simulink model "Sampling_switch_uncertainty"  (R2021b)
settings: Solver=VariableStepAuto  StartTime=0.0  StopTime=10.0  RelTol=1e-3
values from neighbouring files (symbols this model uses):
  bits_number = 13    [launch_pipeline_switch.m]
  cst = 2*pi*fin/1000    [launch_pipeline_switch.m]
  fin = antismear(fin_pre,fs,nfft)    [launch_pipeline_switch.m]
  ts = 1/fs    (= 1)    [launch_pipeline_switch.m]
(part 2 of 2)

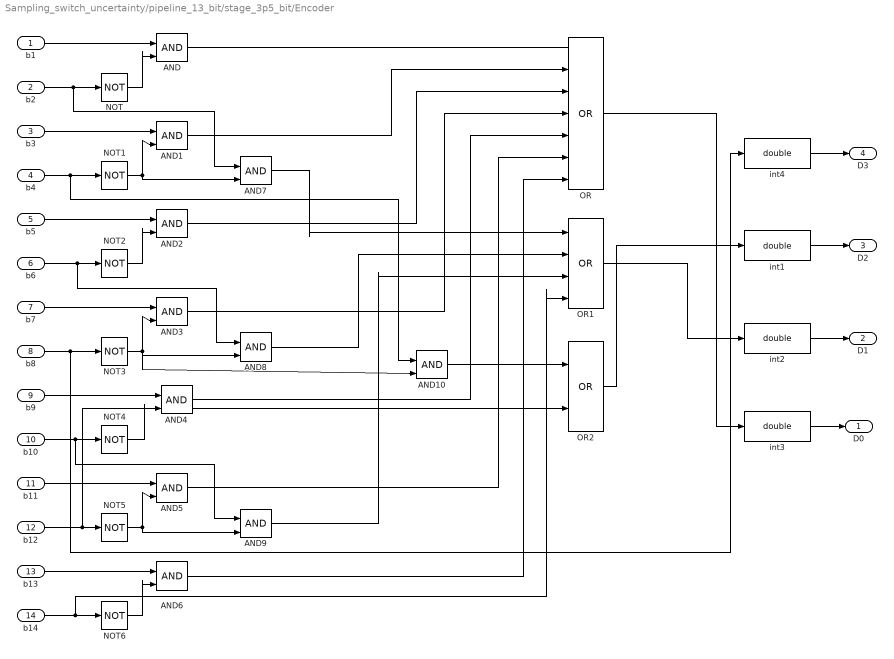
== system Sampling_switch_uncertainty/pipeline_13_bit/stage_3p5_bit/Encoder ==
  b1 : Inport
  b2 : Inport  Port=2
  b3 : Inport  Port=3
  b4 : Inport  Port=4
  b5 : Inport  Port=5
  b6 : Inport  Port=6
  b7 : Inport  Port=7
  b8 : Inport  Port=8
  b9 : Inport  Port=9
  b10 : Inport  Port=10
  b11 : Inport  Port=11
  b12 : Inport  Port=12
  b13 : Inport  Port=13
  b14 : Inport  Port=14
  AND{,1..10} (11 alike) : Logic  IconShape=distinctive  AllPortsSameDT=off  OutDataTypeStr=boolean
  NOT{,1..6} (7 alike) : Logic  Operator=NOT  IconShape=distinctive  AllPortsSameDT=off  OutDataTypeStr=boolean
  OR : Logic  Operator=OR  Inputs=7  IconShape=distinctive  AllPortsSameDT=off  OutDataTypeStr=boolean
  OR1 : Logic  Operator=OR  Inputs=4  IconShape=distinctive  AllPortsSameDT=off  OutDataTypeStr=boolean
  OR2 : Logic  Operator=OR  IconShape=distinctive  AllPortsSameDT=off  OutDataTypeStr=boolean
  int{1..4} (4 alike) : DataTypeConversion  OutDataTypeStr=double
  D0 : Outport
  D1 : Outport  Port=2
  D2 : Outport  Port=3
  D3 : Outport  Port=4
  wires:
  int2/1 -> D1/1
  int3/1 -> D0/1
  int1/1 -> D2/1
  int4/1 -> D3/1
  b14/1 -> OR1/4, NOT6/1
  b12/1 -> OR2/2, NOT5/1
  b10/1 -> AND9/1, NOT4/1
  b8/1 -> int4/1, NOT3/1
  b2/1 -> AND7/1, NOT/1
  b4/1 -> AND10/1, NOT1/1
  b6/1 -> AND8/1, NOT2/1
  b1/1 -> AND/1
  NOT/1 -> AND/2
  b3/1 -> AND1/1
  NOT1/1 -> AND1/2, AND7/2
  b5/1 -> AND2/1
  NOT2/1 -> AND2/2
  b7/1 -> AND3/1
  NOT3/1 -> AND10/2, AND8/2, AND3/2
  b9/1 -> AND4/1
  NOT4/1 -> AND4/2
  b11/1 -> AND5/1
  NOT5/1 -> AND9/2, AND5/2
  b13/1 -> AND6/1
  NOT6/1 -> AND6/2
  OR/1 -> int3/1
  AND/1 -> OR/1
  AND1/1 -> OR/2
  AND2/1 -> OR/3
  AND3/1 -> OR/4
  AND4/1 -> OR/5
  AND5/1 -> OR/6
  AND6/1 -> OR/7
  AND9/1 -> OR1/3
  AND8/1 -> OR1/2
  AND7/1 -> OR1/1
  OR1/1 -> int2/1
  AND10/1 -> OR2/1
  OR2/1 -> int1/1

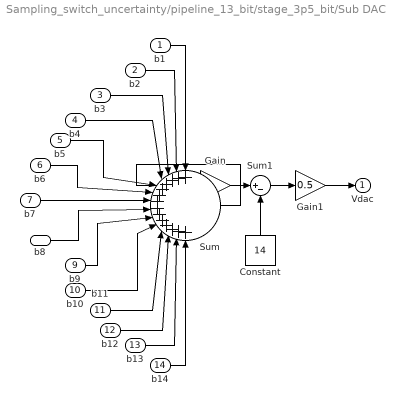
== system Sampling_switch_uncertainty/pipeline_13_bit/stage_3p5_bit/Sub DAC ==
  b1 : Inport
  b2 : Inport  Port=2
  b3 : Inport  Port=3
  b4 : Inport  Port=4
  b5 : Inport  Port=5
  b6 : Inport  Port=6
  b7 : Inport  Port=7
  b8 : Inport  Port=8
  b9 : Inport  Port=9
  b10 : Inport  Port=10
  b11 : Inport  Port=11
  b12 : Inport  Port=12
  b13 : Inport  Port=13
  b14 : Inport  Port=14
  Constant : Constant  Value=14
  Gain : Gain  Gain=2
  Gain1 : Gain  Gain=0.5
  Sum : Sum  Inputs=++++++++++++++
  Sum1 : Sum  Inputs=|+-
  Vdac : Outport
  wires:
  b1/1 -> Sum/1
  b2/1 -> Sum/2
  b3/1 -> Sum/3
  b4/1 -> Sum/4
  b5/1 -> Sum/5
  b6/1 -> Sum/6
  Sum/1 -> Gain/1
  Gain/1 -> Sum1/1
  Constant/1 -> Sum1/2
  Sum1/1 -> Gain1/1
  Gain1/1 -> Vdac/1
  b7/1 -> Sum/7
  b8/1 -> Sum/8
  b9/1 -> Sum/9
  b10/1 -> Sum/10
  b11/1 -> Sum/11
  b12/1 -> Sum/12
  b13/1 -> Sum/13
  b14/1 -> Sum/14
